simulink model "task_1"  (R2024a)
settings: Solver=VariableStepAuto  StartTime=0.0  StopTime=10.0  RelTol=1e-3
settings Model: Creator=bpari  LastModifiedBy=bpari

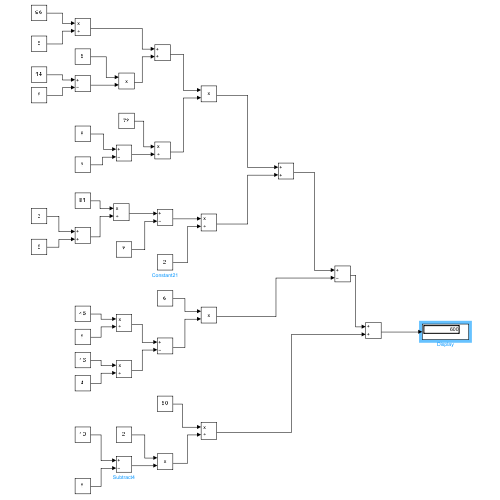
[thumbnail: Simulink's stored preview of the top-level diagram]
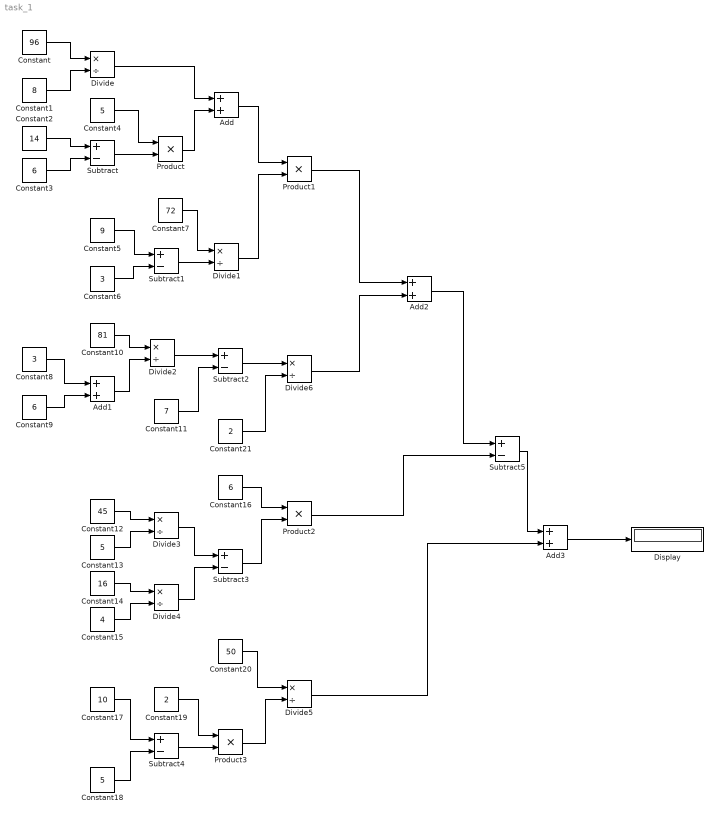
== system task_1 ==
  Add{,1..3} (4 alike) : Sum
  Constant : Constant  Value=96
  Constant1 : Constant  Value=8
  Constant10 : Constant  Value=81
  Constant11 : Constant  Value=7
  Constant12 : Constant  Value=45
  Constant13 : Constant  Value=5
  Constant14 : Constant  Value=16
  Constant15 : Constant  Value=4
  Constant16 : Constant  Value=6
  Constant17 : Constant  Value=10
  Constant18 : Constant  Value=5
  Constant19 : Constant  Value=2
  Constant2 : Constant  Value=14
  Constant20 : Constant  Value=50
  Constant21 : Constant  Value=2
  Constant3 : Constant  Value=6
  Constant4 : Constant  Value=5
  Constant5 : Constant  Value=9
  Constant6 : Constant  Value=3
  Constant7 : Constant  Value=72
  Constant8 : Constant  Value=3
  Constant9 : Constant  Value=6
  Display : Display
  Divide{,1..6} (7 alike) : Product  Inputs=*/  RndMeth=Zero  SaturateOnIntegerOverflow=on
  Product{,1..3} (4 alike) : Product
  Subtract{,1..5} (6 alike) : Sum  Inputs=+-
  wires:
  Constant/1 -> Divide/1
  Constant1/1 -> Divide/2
  Constant2/1 -> Subtract/1
  Constant3/1 -> Subtract/2
  Subtract/1 -> Product/2
  Constant4/1 -> Product/1
  Product/1 -> Add/2
  Divide/1 -> Add/1
  Constant5/1 -> Subtract1/1
  Constant6/1 -> Subtract1/2
  Subtract1/1 -> Divide1/2
  Constant7/1 -> Divide1/1
  Add/1 -> Product1/1
  Divide1/1 -> Product1/2
  Constant8/1 -> Add1/1
  Constant9/1 -> Add1/2
  Add1/1 -> Divide2/2
  Constant10/1 -> Divide2/1
  Divide2/1 -> Subtract2/1
  Constant11/1 -> Subtract2/2
  Constant12/1 -> Divide3/1
  Constant13/1 -> Divide3/2
  Constant15/1 -> Divide4/2
  Constant14/1 -> Divide4/1
  Divide3/1 -> Subtract3/1
  Divide4/1 -> Subtract3/2
  Subtract3/1 -> Product2/2
  Constant16/1 -> Product2/1
  Constant17/1 -> Subtract4/1
  Constant18/1 -> Subtract4/2
  Subtract4/1 -> Product3/2
  Constant19/1 -> Product3/1
  Product3/1 -> Divide5/2
  Constant20/1 -> Divide5/1
  Subtract2/1 -> Divide6/1
  Constant21/1 -> Divide6/2
  Product1/1 -> Add2/1
  Divide6/1 -> Add2/2
  Add2/1 -> Subtract5/1
  Product2/1 -> Subtract5/2
  Subtract5/1 -> Add3/1
  Divide5/1 -> Add3/2
  Add3/1 -> Display/1
